simulink model "ALS_freq3v5"  (Simulink 7.6)
settings: Solver=ode45  StartTime=0.0  StopTime=10.0  RelTol=1e-3
values from neighbouring files (symbols this model uses):
  ArmCavPole = 2*pi* ArmCavFSR / (2* ArmCavFIN)    (= 1178.75567416)    [ALS_lockingv4.m]    (also in ALS_lockingv5.m; ALS_lockingv6.m)
  COMMengaged = 1    [ALS_lockingv4.m]    (also in ALS_lockingv5.m; ALS_lockingv6.m)
  DIFFengaged = 1    [ALS_lockingv4.m]    (also in ALS_lockingv5.m; ALS_lockingv6.m)
  FSSengaged = 1    [ALS_lockingv4.m]    (also in ALS_lockingv5.m; ALS_lockingv6.m)
  gALL = 10^( gALLdB /20)    (= 31622.7766017)    [PDHservo_All_2010_05_21_11_00_19.m]    (also in PDHservo_All_2010_07_19_15_51_34.m = 17500; PMandTMonly_servo.m = 2750)
  gLP = 0    [ALS_lockingv4.m]    (also in ALS_lockingv5.m; ALS_lockingv6.m; PDHservo_All_2010_05_21_11_00_19.m = 1; PDHservo_All_2010_07_19_15_51_34.m = 1)
  gPM = 1    [ALS_lockingv4.m]    (also in ALS_lockingv5.m; ALS_lockingv6.m; PDHservo_All_2010_05_21_11_00_19.m = 0; PDHservo_All_2010_07_19_15_51_34.m = 0)
  gTM = 1    [ALS_lockingv4.m]    (also in ALS_lockingv5.m; ALS_lockingv6.m; PDHservo_All_2010_05_21_11_00_19.m = 0; PDHservo_All_2010_07_19_15_51_34.m = 0)
  gTOP = 0    [ALS_lockingv4.m]    (also in ALS_lockingv5.m; ALS_lockingv6.m; PDHservo_All_2010_05_21_11_00_19.m; PDHservo_All_2010_07_19_15_51_34.m)
  gUIM = 0    [ALS_lockingv4.m]    (also in ALS_lockingv5.m; ALS_lockingv6.m; PDHservo_All_2010_05_21_11_00_19.m; PDHservo_All_2010_07_19_15_51_34.m)
  L_arm = 3995    [ALS_lockingv4.m]    (also in ALS_lockingv5.m; ALS_lockingv6.m)
  nu_IR = cc / lambda_IR    (= 2.81759828947e+14)    [ALS_lockingv4.m]    (also in ALS_lockingv5.m; ALS_lockingv6.m)
  PDHengaged = 1    [ALS_lockingv4.m]    (also in ALS_lockingv5.m; ALS_lockingv6.m)
  prePM = 5e2    (= 500)    [PDHservo_All_2010_05_21_11_00_19.m]    (also in PDHservo_All_2010_07_19_15_51_34.m = 100000; PMandTMonly_servo.m = 70000)
  preUIM = 3e2    (= 300)    [PDHservo_All_2010_05_21_11_00_19.m]    (also in PDHservo_All_2010_07_19_15_51_34.m)
  PSLfrequencyActuator = 1    [ALS_lockingv4.m]    (also in ALS_lockingv5.m; ALS_lockingv6.m)
  RefCavPole = 2*pi * RefCavFSR / (2* RefCavFIN)    (= 470912.891827)    [ALS_lockingv4.m]    (also in ALS_lockingv5.m; ALS_lockingv6.m)
  TTFSSengaged = 1    [ALS_lockingv4.m]    (also in ALS_lockingv5.m; ALS_lockingv6.m)
  uPZT_local = 3e6    (= 3000000)    [ALS_lockingv4.m]    (also in ALS_lockingv5.m; ALS_lockingv6.m)
libraries: cstblocks x22
settings Model: Creator=slagmolen  LastModifiedBy=slagmolen
settings DebuggingCC: SolverPrmCheckMsg=none  StrictBusMsg=Warning
settings SFSimCC: SimParseCustomCode=off

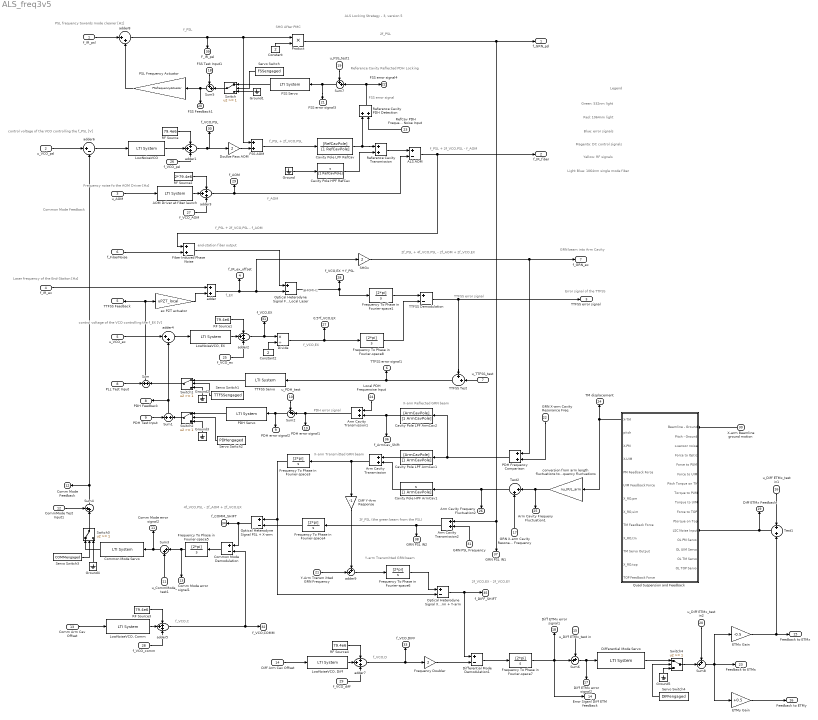
== system ALS_freq3v5 ==
  note: PSL frequency towards
      | mode cleaner [Hz]
  note: SHG After PMC
  note: f_PSL
  note: f_PSL + 2f_VCO,PSL
  note: f_AOM
  note: f_PSL + 2f_VCO,PSL - f_AOM
  note: f_PSL + 2f_VCO,PSL - f_AOM
  note: f_VCO,EX
  note: f_EX
  note: TTFSS error signal
  note: 2f_PSL
  note: end-station
      | fiber output
  note: @40MHz
  note: control voltage of the VCO
      | controlling the f_PSL [V]
  note: Frequency noise fo the
      | AOM Driver [Hz]
  note: Laser frequency of the
      | End-Staiton [Hz]
  note: Error signal of the
      | TTFSS
  note: control voltage of the VCO
      | controlling the f_EX [V]
  note: 2f_PSL + 4f_VCO,PSL - 2f_AOM + 2f_VCO,EX
  note: GRN beam into
      | Arm Cavity
  note: PDH error signal
  note: 2f_PSL (the green beam from the PSL)
  note: X-arm Transmitted GRN beam
  note: f_VCO,C
  note: 4f_VCO,PSL - 2f_AOM + 2f_VCO,EX
  note: Y-arm Transmitted GRN beam
  note: f_VCO,D
  note: 2f_VCO,EX - 2f_VCO,EY
  note: X-arm Reflected GRN beam
  note: FSS error signal
  note: Reference Cavity Reflected PDH Locking
  note: Common Mode Feedback
  note: ALS Locking Strategy - 3, version 5
  note: Green: 532nm light
  note: Red: 1064nm light
  note: Blue: error signals
  note: Magenta: DC control signals
  note: Yellow: RF signals
  note: Light Blue: 1064nm single mode fiber
  note: Legend
  f_IR_psl : Inport
  u_VCO_psl : Inport  Port=2
  u_AOM : Inport  Port=3
  f_IR_ex : Inport  Port=4
  u_VCO_ex : Inport  Port=5
  f_FiberNoise : Inport  Port=6
  u_TTFSS_test : Inport  Port=7
  PLL Test Input : Inport  Port=8
  PDH Test Input : Inport  Port=9
  u_PDH_test : Inport  Port=10
  u_CommMode_test1 : Inport  Port=11
  CommMode Test Input1 : Inport  Port=12
  Comm Arm Cav Offset : Inport  Port=13
  Diff Arm Cav Offset : Inport  Port=14
  u_Diff ETMx_test in : Inport  Port=15
  u_Diff ETMx_test in1 : Inport  Port=16
  GRN X-arm Cavity Resonance Frequency : Inport  Port=17
  FSS Test Input1 : Inport  Port=18
  u_FSS_test1 : Inport  Port=19
  u_Diff ETMx_test in2 : Inport  Port=20
  Y-Arm Transm itted GRN Frequency : Inport  Port=21
  GRN X-arm Cavity Resonance Freq : Inport  Port=22
  RefCav PDH Frequency Noise Input : Inport  Port=23
  Local PDH Frequenoise Input : Inport  Port=24
  f_VCO_ex : Inport  Port=25
  f_VCO_psl : Inport  Port=26
  f_VCO_AOM : Inport  Port=27
  f_VCO_comm : Inport  Port=28
  f_VCO_diff : Inport  Port=29
  X-arm Beamline ground motion : Inport  Port=30
  GRN PSL Frequency : Inport  Port=31
  " Test1" : Sum  Inputs=+|+
  " Test2" : Sum  Inputs=|++
  ALS AOM : Sum  Inputs=+-
  AOM Driver at fiber launch : cstblocks/LTI System  SystemSampleTime=-1  sys=AOM_Driver  IC=[]
  Arm Cavity Transmission : Sum
  Arm Cavity Transmission1 : Sum
  Arm Cavity Transmission2 : Sum
  Cavity Pole HPF ArmCav1 : TransferFcn  Numerator=[1 0]  Denominator=[1 ArmCavPole]
  Cavity Pole HPF RefCav : TransferFcn  Numerator=[1 0]  Denominator=[1 RefCavPole]
  Cavity Pole LPF ArmCav1 : TransferFcn  Numerator=[ArmCavPole]  Denominator=[1 ArmCavPole]
  Cavity Pole LPF ArmCav2 : TransferFcn  Numerator=[ArmCavPole]  Denominator=[1 ArmCavPole]
  Cavity Pole LPF RefCav : TransferFcn  Numerator=[RefCavPole]  Denominator=[1 RefCavPole]
  Common Mode Demodulation : Sum  Inputs=+-
  Common Mode Servo : cstblocks/LTI System  SystemSampleTime=-1  sys=CommonMode_Servo  IC=[]
  Constant : Constant  Value=2
  Constant2 : Constant  Value=2
  Diff Y-Arm Response : Gain  Gain=-1
  Differential Mode Demodulation1 : Sum  Inputs=+-
  Differential Mode Servo : cstblocks/LTI System  SystemSampleTime=-1  sys=DifferentialMode_Servo  IC=[]
  Divide : Product  Inputs=*/
  Doulbe Pass AOM : Gain  Gain=2
  ETMx Gain : Gain  Gain=-0.5
  ETMy Gain : Gain  Gain=+0.5
  FSS AOM : Sum
  FSS Servo : cstblocks/LTI System  SystemSampleTime=-1  sys=FSS_Servo  IC=[]
  Fiber Induced Phase Noise : Sum
  Frequency Doubler : Gain  Gain=2
  Frequency To Phase in Fourier-space{1,3..8} (7 alike) : TransferFcn  Numerator=[2*pi]  Denominator=[1 0]
  Ground{,1..5} (6 alike) : Ground
  LowNoiseVCO : cstblocks/LTI System  SystemSampleTime=-1  sys=LowNoiseVCO_psl  IC=[]
  "LowNoiseVCO, Comm" : cstblocks/LTI System  SystemSampleTime=-1  sys=LowNoiseVCO_comm  IC=[]
  "LowNoiseVCO, Diff" : cstblocks/LTI System  SystemSampleTime=-1  sys=LowNoiseVCO_diff  IC=[]
  "LowNoiseVCO, EX" : cstblocks/LTI System  SystemSampleTime=-1  sys=LowNoiseVCO_local  IC=[]
  Optical Heterodyne Signal Fiber Output + Local Laser : Sum  Inputs=+-
  Optical Heterodyne Signal PSL + X-arm : Sum  Inputs=+-
  Optical Heterodyne Signal X-arm + Y-arm : Sum  Inputs=+-
  PDH Frequency Comparison : Sum
  PDH Servo : cstblocks/LTI System  SystemSampleTime=-1  sys=PDH_Servo  IC=[]
  PSL Frequency Actuator : Gain  Gain=PSLfrequencyActuator
  Product : Product  RndMeth=Zero
  Quad Suspension and Feedback : Subsystem
  RF Source{,1,3..4} (4 alike) : Constant  Value=79.4e6
  RF Source2 : Constant  Value=2*79.4e6
  Reference Cavity PDH Detection : Sum
  Reference Cavity Transmission : Sum
  SHGx : Gain  Gain=2
  Servo Switch : Constant  Value=FSSengaged
  Servo Switch1 : Constant  Value=TTFSSengaged
  Servo Switch2 : Constant  Value=PDHengaged
  Servo Switch3 : Constant  Value=COMMengaged
  Servo Switch4 : Constant  Value=DIFFengaged
  Sum : Sum  Inputs=+|+
  Sum1 : Sum  Inputs=+|+
  Sum{2,4..8} (6 alike) : Sum  Inputs=++|
  Sum3 : Sum  Inputs=|++
  Switch{,1..4} (5 alike) : Switch  Threshold=1
  TTFSS Demodulation : Sum  Inputs=+-
  TTFSS Servo : cstblocks/LTI System  SystemSampleTime=-1  sys=TTFSS_Servo  IC=[]
  TTFSS Test : Sum  Inputs=++|
  adder : Sum
  adder{1..3,5,7} (5 alike) : Sum  Inputs=+++
  adder4 : Sum  Inputs=|++
  adder6 : Sum  Inputs=|+-
  adder8 : Sum  Inputs=|++
  adder9 : Sum  Inputs=++|
  conversion from arm length fluctuations to frequency fluctuations : Gain  Gain=nu_IR/L_arm
  ex PZT actuator : Gain  Gain=uPZT_local
  f_GRN_psl : Outport
  f_IR_fiber : Outport  Port=2
  TTFSS error signal : Outport  Port=3
  f_IR_ex_offset : Outport  Port=4
  TTFSS Feedback : Outport  Port=5
  TTFSS error signal1 : Outport  Port=6
  f_GRN_ex : Outport  Port=7
  PDH Feedback : Outport  Port=8
  PDH error signal2 : Outport  Port=9
  PDH error signal1 : Outport  Port=10
  Comm Mode error signal2 : Outport  Port=11
  Comm Mode Feedback : Outport  Port=12
  Comm Mode error signal1 : Outport  Port=13
  Error Siganl Diff ETM feedback : Outport  Port=14
  Feedback to ETMx : Outport  Port=15
  Feedback to ETMy : Outport  Port=16
  Diff ETMx error signal2 : Outport  Port=17
  Diff ETMx error signal1 : Outport  Port=18
  Diff ETMx Feedback : Outport  Port=19
  FSS Feedback1 : Outport  Port=20
  FSS error signal3 : Outport  Port=21
  FSS error signal4 : Outport  Port=22
  Feedback to ETMs : Outport  Port=23
  TM displacement : Outport  Port=24
  Arm Cavity Frequeny Fluctuation1 : Outport  Port=25
  Arm Cavity Frequeny Fluctuation2 : Outport  Port=26
  0.5*f_VCO,EX : Outport  Port=27
  f_VCO,EX + f_PSL : Outport  Port=28
  f_AOM : Outport  Port=29
  f_VCO,PSL : Outport  Port=30
  f_VCO,EX : Outport  Port=31
  f_VCO,COMM : Outport  Port=32
  f_VCO,DIFF : Outport  Port=33
  f_COMM_SHIFT : Outport  Port=34
  f_DIFF_SHIFT : Outport  Port=35
  f_ArmCav_Shift : Outport  Port=36
  GRN PSL IN1 : Outport  Port=37
  GRN PSL IN2 : Outport  Port=38
  F_IR_psl : Outport  Port=39
  wires:
  Constant/1 -> Product/2
  Product/1 -> f_GRN_psl/1, Arm Cavity Transmission2/1, GRN PSL IN1/1
  Doulbe Pass AOM/1 -> FSS AOM/2
  FSS AOM/1 -> Cavity Pole LPF RefCav/1
  Cavity Pole LPF RefCav/1 -> Reference Cavity Transmission/1, Reference Cavity PDH Detection/1
  Cavity Pole HPF RefCav/1 -> Reference Cavity Transmission/2
  u_AOM/1 -> AOM Driver at fiber launch/1
  Reference Cavity Transmission/1 -> ALS AOM/1
  ALS AOM/1 -> f_IR_fiber/1, Fiber Induced Phase Noise/1
  f_FiberNoise/1 -> Fiber Induced Phase Noise/2
  Constant2/1 -> Divide/2
  ex PZT actuator/1 -> adder/2
  TTFSS Demodulation/1 -> TTFSS error signal/1, TTFSS Test/1
  LowNoiseVCO/1 -> adder1/2
  adder1/1 -> Doulbe Pass AOM/1, f_VCO,PSL/1
  RF Source/1 -> adder1/1
  RF Source1/1 -> adder2/1
  "LowNoiseVCO, EX"/1 -> adder2/2
  adder2/1 -> Divide/1, f_VCO,EX/1
  RF Source2/1 -> adder3/1
  AOM Driver at fiber launch/1 -> adder3/2
  adder3/1 -> ALS AOM/2, f_AOM/1
  adder/1 -> f_IR_ex_offset/1, SHGx/1, Optical Heterodyne Signal Fiber Output + Local Laser/2
  TTFSS Test/1 -> TTFSS Servo/1, TTFSS error signal1/1
  u_TTFSS_test/1 -> TTFSS Test/2
  SHGx/1 -> f_GRN_ex/1, PDH Frequency Comparison/1
  PLL Test Input/1 -> Sum/1
  Sum/1 -> ex PZT actuator/1, TTFSS Feedback/1
  Cavity Pole LPF ArmCav1/1 -> Arm Cavity Transmission/1
  Cavity Pole HPF ArmCav1/1 -> Arm Cavity Transmission/2
  Arm Cavity Transmission/1 -> Frequency To Phase in Fourier-space3/1, Diff Y-Arm Response/1
  adder4/1 -> "LowNoiseVCO, EX"/1
  u_VCO_ex/1 -> adder4/1
  Sum1/1 -> adder4/2, PDH Feedback/1
  PDH Test Input/1 -> Sum1/1
  Sum2/1 -> PDH Servo/1, PDH error signal2/1
  u_PDH_test/1 -> Sum2/1
  Frequency To Phase in Fourier-space3/1 -> Optical Heterodyne Signal PSL + X-arm/1, Optical Heterodyne Signal X-arm + Y-arm/2
  Frequency To Phase in Fourier-space4/1 -> Optical Heterodyne Signal PSL + X-arm/2
  RF Source3/1 -> adder5/1
  "LowNoiseVCO, Comm"/1 -> adder5/2
  adder5/1 -> Common Mode Demodulation/2, f_VCO,COMM/1
  u_VCO_psl/1 -> adder6/1
  adder6/1 -> LowNoiseVCO/1
  Common Mode Demodulation/1 -> Frequency To Phase in Fourier-space5/1
  Sum3/1 -> Common Mode Servo/1, Comm Mode error signal2/1
  u_CommMode_test1/1 -> Sum3/2
  Sum4/1 -> adder6/2, Comm Mode Feedback/1
  CommMode Test Input1/1 -> Sum4/1
  Comm Arm Cav Offset/1 -> "LowNoiseVCO, Comm"/1
  Optical Heterodyne Signal PSL + X-arm/1 -> Common Mode Demodulation/1, f_COMM_SHIFT/1
  Frequency To Phase in Fourier-space6/1 -> Optical Heterodyne Signal X-arm + Y-arm/1
  RF Source4/1 -> adder7/1
  "LowNoiseVCO, Diff"/1 -> adder7/2
  adder7/1 -> Frequency Doubler/1, f_VCO,DIFF/1
  Diff Arm Cav Offset/1 -> "LowNoiseVCO, Diff"/1
  Optical Heterodyne Signal X-arm + Y-arm/1 -> Differential Mode Demodulation1/1, f_DIFF_SHIFT/1
  Frequency Doubler/1 -> Differential Mode Demodulation1/2
  ETMy Gain/1 -> Feedback to ETMy/1
  f_IR_ex/1 -> adder/1
  u_Diff ETMx_test in/1 -> Sum6/1
  " Test1"/1 -> Diff ETMx Feedback/1, Quad Suspension and Feedback/12(LSC Noise Input)
  u_Diff ETMx_test in1/1 -> " Test1"/1
  PDH Frequency Comparison/1 -> Cavity Pole LPF ArmCav1/1, Cavity Pole LPF ArmCav2/1
  ETMx Gain/1 -> " Test1"/2, Feedback to ETMx/1
  Sum5/1 -> FSS Feedback1/1, PSL Frequency Actuator/1
  FSS Test Input1/1 -> Sum5/1
  Sum7/1 -> FSS Servo/1, FSS error signal3/1
  u_FSS_test1/1 -> Sum7/1
  PSL Frequency Actuator/1 -> adder8/2
  adder8/1 -> Product/1, FSS AOM/1, F_IR_psl/1
  f_IR_psl/1 -> adder8/1
  Sum6/1 -> Diff ETMx error signal2/1, Differential Mode Servo/1
  u_Diff ETMx_test in2/1 -> Sum8/1
  Sum8/1 -> ETMx Gain/1, ETMy Gain/1, Feedback to ETMs/1
  Ground/1 -> Cavity Pole HPF RefCav/1
  " Test2"/1 -> Arm Cavity Frequeny Fluctuation2/1, Cavity Pole HPF ArmCav1/1
  GRN X-arm Cavity Resonance Freq/1 -> PDH Frequency Comparison/2
  adder9/1 -> Frequency To Phase in Fourier-space6/1
  Y-Arm Transm itted GRN Frequency/1 -> adder9/2
  Diff Y-Arm Response/1 -> adder9/1
  Quad Suspension and Feedback/1(X-TM) -> conversion from arm length fluctuations to frequency fluctuations/1, TM displacement/1
  conversion from arm length fluctuations to frequency fluctuations/1 -> " Test2"/1, Arm Cavity Frequeny Fluctuation1/1
  GRN X-arm Cavity Resonance Frequency/1 -> " Test2"/2
  Reference Cavity PDH Detection/1 -> Sum7/2, FSS error signal4/1
  RefCav PDH Frequency Noise Input/1 -> Reference Cavity PDH Detection/2
  Arm Cavity Transmission1/1 -> Sum2/2, PDH error signal1/1
  Cavity Pole LPF ArmCav2/1 -> Arm Cavity Transmission1/2, f_ArmCav_Shift/1
  Local PDH Frequenoise Input/1 -> Arm Cavity Transmission1/1
  Ground1/1 -> Switch/3
  Servo Switch/1 -> Switch/2
  Switch/1 -> Sum5/2
  FSS Servo/1 -> Switch/1
  Servo Switch1/1 -> Switch1/2
  TTFSS Servo/1 -> Switch1/1
  Ground2/1 -> Switch1/3
  Switch1/1 -> Sum/2
  Servo Switch2/1 -> Switch2/2
  PDH Servo/1 -> Switch2/1
  Switch2/1 -> Sum1/2
  Ground3/1 -> Switch2/3
  Switch3/1 -> Sum4/2
  Common Mode Servo/1 -> Switch3/1
  Ground4/1 -> Switch3/3
  Servo Switch3/1 -> Switch3/2
  Switch4/1 -> Sum8/2
  Differential Mode Servo/1 -> Switch4/1
  Ground5/1 -> Switch4/3
  Servo Switch4/1 -> Switch4/2
  Fiber Induced Phase Noise/1 -> Optical Heterodyne Signal Fiber Output + Local Laser/1
  Divide/1 -> 0.5*f_VCO,EX/1, Frequency To Phase in Fourier-space8/1
  Optical Heterodyne Signal Fiber Output + Local Laser/1 -> f_VCO,EX + f_PSL/1, Frequency To Phase in Fourier-space1/1
  Differential Mode Demodulation1/1 -> Frequency To Phase in Fourier-space7/1
  Frequency To Phase in Fourier-space7/1 -> Sum6/2, Diff ETMx error signal1/1, Error Siganl Diff ETM feedback/1
  Frequency To Phase in Fourier-space5/1 -> Sum3/1, Comm Mode error signal1/1
  Frequency To Phase in Fourier-space8/1 -> TTFSS Demodulation/2
  Frequency To Phase in Fourier-space1/1 -> TTFSS Demodulation/1
  f_VCO_ex/1 -> adder2/3
  f_VCO_psl/1 -> adder1/3
  f_VCO_AOM/1 -> adder3/3
  f_VCO_comm/1 -> adder5/3
  f_VCO_diff/1 -> adder7/3
  X-arm Beamline ground motion/1 -> Quad Suspension and Feedback/1(Beamline - Ground)
  Arm Cavity Transmission2/1 -> Frequency To Phase in Fourier-space4/1, GRN PSL IN2/1
  GRN PSL Frequency/1 -> Arm Cavity Transmission2/2

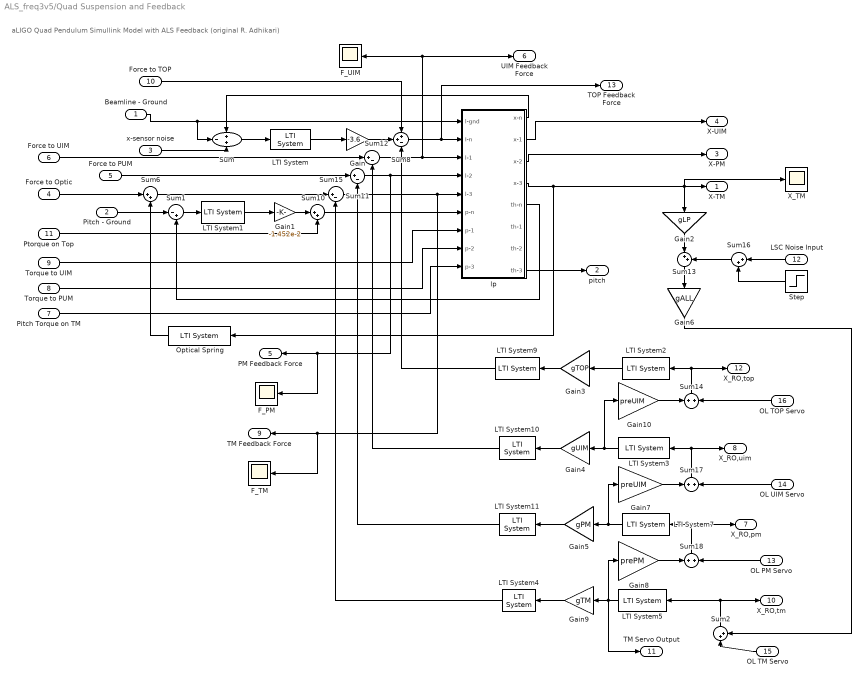
== system ALS_freq3v5/Quad Suspension and Feedback ==
  note: aLIGO Quad Pendulum Simullink Model
      | with ALS Feedback
      | (original  R. Adhikari)
  Beamline - Ground : Inport
  Pitch - Ground : Inport  Port=2
  x-sensor noise : Inport  Port=3
  Force to Optic : Inport  Port=4
  Force to PUM : Inport  Port=5
  Force to UIM : Inport  Port=6
  Pitch Torque on TM : Inport  Port=7
  Torque to PUM : Inport  Port=8
  Torque to UIM : Inport  Port=9
  Force to TOP : Inport  Port=10
  Ptorque on Top : Inport  Port=11
  LSC Noise Input : Inport  Port=12
  OL PM Servo : Inport  Port=13
  OL UIM Servo : Inport  Port=14
  OL TM Servo : Inport  Port=15
  OL TOP Servo : Inport  Port=16
  F_PM : Scope
      settings: TimeRange=10
  F_TM : Scope
      settings: TimeRange=20  SaveName=ScopeData2
  F_UIM : Scope
      settings: TimeRange=10  SaveName=ScopeData3
  Gain : Gain  Gain=-3.6  OutDataTypeStr=Inherit: Same as input  ParamDataTypeStr=Inherit: Same as input
  Gain1 : Gain  Gain=-1.452e-2  OutDataTypeStr=Inherit: Same as input  ParamDataTypeStr=Inherit: Same as input
  Gain10 : Gain  Gain=preUIM
  Gain2 : Gain  Gain=gLP  OutDataTypeStr=Inherit: Same as input  ParamDataTypeStr=Inherit: Same as input
  Gain3 : Gain  Gain=gTOP
  Gain4 : Gain  Gain=gUIM
  Gain5 : Gain  Gain=gPM
  Gain6 : Gain  Gain=gALL
  Gain7 : Gain  Gain=preUIM
  Gain8 : Gain  Gain=prePM
  Gain9 : Gain  Gain=gTM
  LTI System : cstblocks/LTI System  SystemSampleTime=-1  sys=ldamp  IC=[]
  LTI System1 : cstblocks/LTI System  SystemSampleTime=-1  sys=pdamp  IC=[]
  LTI System10 : cstblocks/LTI System  SystemSampleTime=-1  sys=coUIM  IC=[]
  LTI System11 : cstblocks/LTI System  SystemSampleTime=-1  sys=coPM  IC=[]
  LTI System2 : cstblocks/LTI System  SystemSampleTime=-1  sys=ServoTOP  IC=[]
  LTI System3 : cstblocks/LTI System  SystemSampleTime=-1  sys=ServoUIM  IC=[]
  LTI System4 : cstblocks/LTI System  SystemSampleTime=-1  sys=coTM  IC=[]
  LTI System5 : cstblocks/LTI System  SystemSampleTime=-1  sys=ServoTM  IC=[]
  LTI System7 : cstblocks/LTI System  SystemSampleTime=-1  sys=ServoPM  IC=[]
  LTI System9 : cstblocks/LTI System  SystemSampleTime=-1  sys=coTOP  IC=[]
  Optical Spring : cstblocks/LTI System  SystemSampleTime=-1  sys=k_ospring  IC=[]
  Step : Step  SampleTime=0
  Sum : Sum  Inputs=+-+  InputSameDT=on  OutDataTypeStr=Inherit: Same as first input
  Sum1 : Sum  Inputs=|-+  InputSameDT=on  OutDataTypeStr=Inherit: Same as first input
  Sum{2,6,10,13,16} (5 alike) : Sum  Inputs=|++  InputSameDT=on  OutDataTypeStr=Inherit: Same as first input
  Sum11 : Sum  Inputs=|+-  InputSameDT=on  OutDataTypeStr=Inherit: Same as first input
  Sum12 : Sum  Inputs=|+-  InputSameDT=on  OutDataTypeStr=Inherit: Same as first input
  Sum14 : Sum  Inputs=+|+  InputSameDT=on  OutDataTypeStr=Inherit: Same as first input
  Sum15 : Sum  Inputs=|+-  InputSameDT=on  OutDataTypeStr=Inherit: Same as first input
  Sum17 : Sum  Inputs=+|+  InputSameDT=on  OutDataTypeStr=Inherit: Same as first input
  Sum18 : Sum  Inputs=+|+  InputSameDT=on  OutDataTypeStr=Inherit: Same as first input
  Sum8 : Sum  Inputs=++-  InputSameDT=on  OutDataTypeStr=Inherit: Same as first input
  X_TM : Scope
      settings: TimeRange=20
  lp : Subsystem
  X-TM : Outport
  pitch : Outport  Port=2
  X-PM : Outport  Port=3
  X-UIM : Outport  Port=4
  PM Feedback Force : Outport  Port=5
  UIM Feedback Force : Outport  Port=6
  X_RO,pm : Outport  Port=7
  X_RO,uim : Outport  Port=8
  TM Feedback Force : Outport  Port=9
  X_RO,tm : Outport  Port=10
  TM Servo Output : Outport  Port=11
  X_RO,top : Outport  Port=12
  TOP Feedback Force : Outport  Port=13
  wires:
  Gain1/1 -> Sum10/1
  lp/5(th-n) -> Sum1/2
  lp/1(x-n) -> Sum/1
  LTI System/1 -> Gain/1
  Sum1/1 -> LTI System1/1
  Sum/1 -> LTI System/1
  Pitch - Ground/1 -> Sum1/1
  lp/4(x-3) -> Optical Spring/1, X-TM/1, Gain2/1, X_TM/1
  lp/8(th-3) -> pitch/1
  LTI System1/1 -> Gain1/1
  x-sensor noise/1 -> Sum/3
  Pitch Torque on TM/1 -> lp/9(p-3)
  Torque to PUM/1 -> lp/8(p-2)
  Torque to UIM/1 -> lp/7(p-1)
  Force to Optic/1 -> Sum6/1
  Optical Spring/1 -> Sum6/2
  Gain/1 -> Sum8/2
  Sum8/1 -> lp/2(I-n), TOP Feedback Force/1
  Force to TOP/1 -> Sum8/1
  Sum10/1 -> lp/6(p-n)
  Ptorque on Top/1 -> Sum10/2
  lp/3(x-2) -> X-PM/1
  lp/2(x-1) -> X-UIM/1
  Sum11/1 -> lp/4(l-2), PM Feedback Force/1, F_PM/1
  Force to PUM/1 -> Sum11/1
  Sum12/1 -> lp/3(l-1), UIM Feedback Force/1, F_UIM/1
  Force to UIM/1 -> Sum12/1
  Beamline - Ground/1 -> Sum/2, lp/1(l-gnd)
  Sum6/1 -> Sum15/1
  Sum15/1 -> lp/5(l-3), TM Feedback Force/1, F_TM/1
  LSC Noise Input/1 -> Sum16/1
  Sum16/1 -> Sum13/2
  Step/1 -> Sum16/2
  Sum13/1 -> Gain6/1
  Gain2/1 -> Sum13/1
  Sum2/1 -> LTI System5/1, X_RO,tm/1
  OL TM Servo/1 -> Sum2/1
  Gain6/1 -> Sum2/2
  Sum18/1 -> LTI System7/1, X_RO,pm/1
  OL PM Servo/1 -> Sum18/2
  Sum17/1 -> LTI System3/1, X_RO,uim/1
  OL UIM Servo/1 -> Sum17/2
  Sum14/1 -> LTI System2/1, X_RO,top/1
  OL TOP Servo/1 -> Sum14/2
  Gain5/1 -> LTI System11/1
  LTI System7/1 -> Gain5/1, Gain7/1
  LTI System11/1 -> Sum11/2
  LTI System10/1 -> Sum12/2
  Gain4/1 -> LTI System10/1
  LTI System9/1 -> Sum8/3
  LTI System5/1 -> Gain9/1, Gain8/1, TM Servo Output/1
  Gain9/1 -> LTI System4/1
  LTI System4/1 -> Sum15/2
  LTI System3/1 -> Gain4/1, Gain10/1
  LTI System2/1 -> Gain3/1
  Gain3/1 -> LTI System9/1
  Gain7/1 -> Sum17/1
  Gain8/1 -> Sum18/1
  Gain10/1 -> Sum14/1

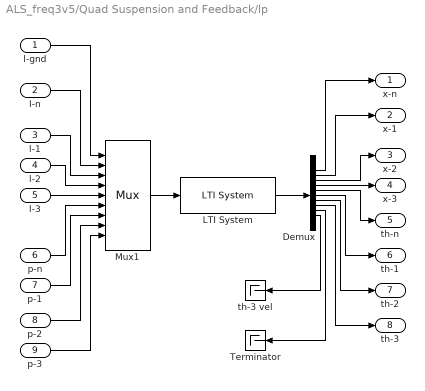
== system ALS_freq3v5/Quad Suspension and Feedback/lp ==
  l-gnd : Inport
  I-n : Inport  Port=2
  l-1 : Inport  Port=3
  l-2 : Inport  Port=4
  l-3 : Inport  Port=5
  p-n : Inport  Port=6
  p-1 : Inport  Port=7
  p-2 : Inport  Port=8
  p-3 : Inport  Port=9
  Demux : Demux  Outputs=10
  LTI System : cstblocks/LTI System  SystemSampleTime=-1  sys=lpe  IC=[0]
  Mux1 : Mux  Inputs=9
      settings: DisplayOption=signals
  Terminator : Terminator
  th-3 vel : Terminator
  x-n : Outport
  x-1 : Outport  Port=2
  x-2 : Outport  Port=3
  x-3 : Outport  Port=4
  th-n : Outport  Port=5
  th-1 : Outport  Port=6
  th-2 : Outport  Port=7
  th-3 : Outport  Port=8
  wires:
  Mux1/1 -> LTI System/1
  LTI System/1 -> Demux/1
  Demux/1 -> x-n/1
  Demux/2 -> x-1/1
  Demux/3 -> x-2/1
  Demux/4 -> x-3/1
  Demux/5 -> th-n/1
  Demux/6 -> th-1/1
  Demux/7 -> th-2/1
  Demux/8 -> th-3/1
  l-gnd/1 -> Mux1/1
  I-n/1 -> Mux1/2
  l-1/1 -> Mux1/3
  l-2/1 -> Mux1/4
  l-3/1 -> Mux1/5
  p-n/1 -> Mux1/6
  p-1/1 -> Mux1/7
  p-2/1 -> Mux1/8
  p-3/1 -> Mux1/9
  Demux/9 -> Terminator/1
  Demux/10 -> th-3 vel/1
